simulink model "simulation"  (R2021b)
settings: Solver=VariableStepAuto  StartTime=0.0  StopTime=50  RelTol=1e-3
values from neighbouring files (symbols this model uses):
  g = 9.8    [script.m]
  l = 1    [script.m]
  m = 1    [script.m]
libraries: spsRMSLib x1
settings Model: Creator=mehdi  LastModifiedBy=mehdi

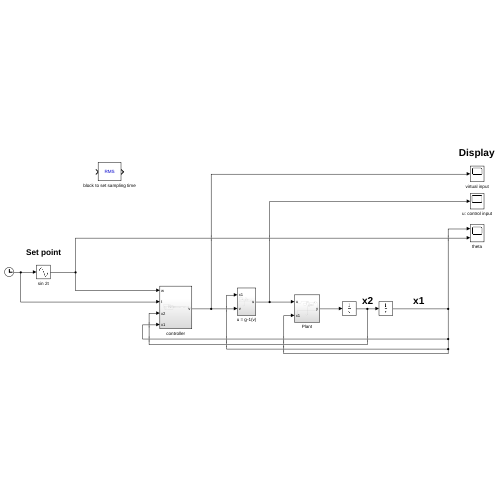
[thumbnail: Simulink's stored preview of the top-level diagram]
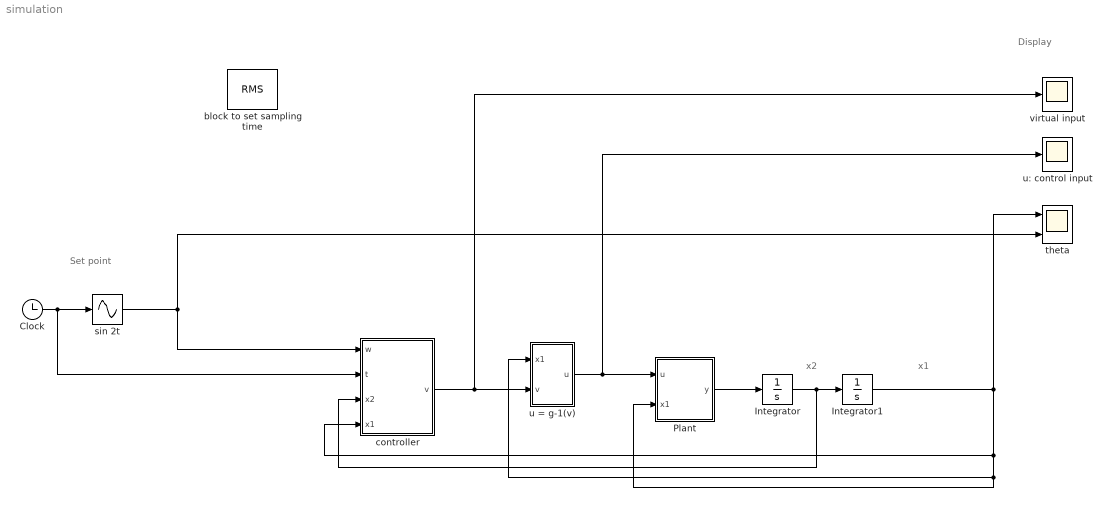
== system simulation ==
  note: Display
  note: x2
  note: Set point
  note: x1
  Clock : Clock
  Integrator : Integrator  ContinuousStateAttributes='omega'
  Integrator1 : Integrator  ContinuousStateAttributes='theta'
  Plant : Subsystem
  block to set sampling time : spsRMSLib/RMS  TrueRMS=on  Freq=60  RMSInit=120  Ts=0.001
  controller : Subsystem
  sin 2t : Sin  TimeSource=Use external signal  Frequency=2  SampleTime=0
  theta : Scope  NumInputPorts=2
  u = g-1(v) : Subsystem
  u: control input : Scope
  virtual input : Scope
  wires:
  Integrator/1 -> Integrator1/1, controller/3(x2)
  Integrator1/1 -> theta/1, Plant/2(x1), u = g-1(v)/1(x1), controller/4(x1)
  Clock/1 -> sin 2t/1, controller/2(t)
  sin 2t/1 -> theta/2, controller/1(w)
  controller/1(v) -> virtual input/1, u = g-1(v)/2(v)
  u = g-1(v)/1(u) -> u: control input/1, Plant/1(u)
  Plant/1(y) -> Integrator/1

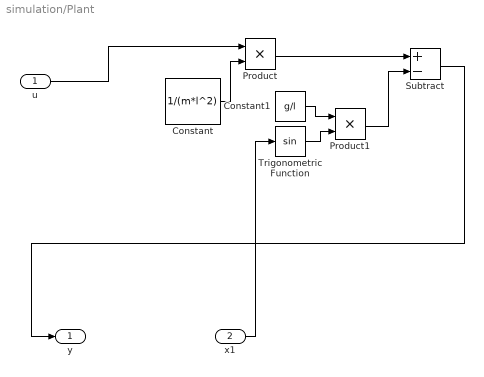
== system simulation/Plant ==
  u : Inport
  x1 : Inport  Port=2
  Constant : Constant  Value=1/(m*l^2)
  Constant1 : Constant  Value=g/l
  Product : Product
  Product1 : Product
  Subtract : Sum  Inputs=+-
  Trigonometric Function : Trigonometry
  y : Outport
  wires:
  u/1 -> Product/1
  Subtract/1 -> y/1
  Product/1 -> Subtract/1
  Constant1/1 -> Product1/1
  Constant/1 -> Product/2
  Product1/1 -> Subtract/2
  x1/1 -> Trigonometric Function/1
  Trigonometric Function/1 -> Product1/2

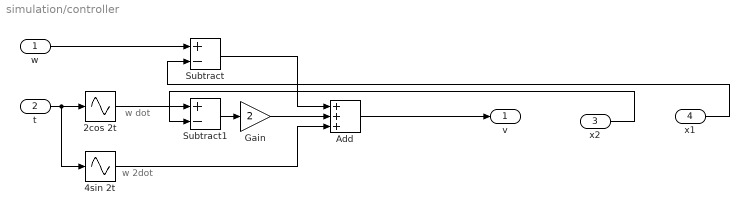
== system simulation/controller ==
  note: w 2dot
  note: w dot
  w : Inport
  t : Inport  Port=2
  x2 : Inport  Port=3
  x1 : Inport  Port=4
  2cos 2t : Sin  TimeSource=Use external signal  Amplitude=2  Frequency=2  Phase=90  SampleTime=0
  4sin 2t : Sin  TimeSource=Use external signal  Amplitude=-4  Frequency=2  SampleTime=0
  Add : Sum  Inputs=+++
  Gain : Gain  Gain=2
  Subtract : Sum  Inputs=+-
  Subtract1 : Sum  Inputs=+-
  v : Outport
  wires:
  4sin 2t/1 -> Add/3
  w/1 -> Subtract/1
  Subtract1/1 -> Gain/1
  t/1 -> 4sin 2t/1, 2cos 2t/1
  Gain/1 -> Add/2
  x1/1 -> Subtract/2
  Subtract/1 -> Add/1
  x2/1 -> Subtract1/2
  2cos 2t/1 -> Subtract1/1
  Add/1 -> v/1

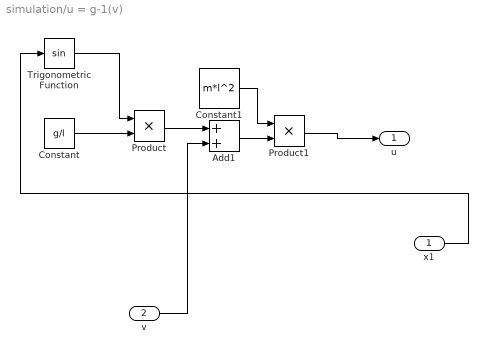
== system simulation/u = g-1(v) ==
  x1 : Inport
  v : Inport  Port=2
  Add1 : Sum
  Constant : Constant  Value=g/l
  Constant1 : Constant  Value=m*l^2
  Product : Product
  Product1 : Product
  Trigonometric Function : Trigonometry
  u : Outport
  wires:
  Product/1 -> Add1/1
  Add1/1 -> Product1/2
  v/1 -> Add1/2
  Product1/1 -> u/1
  Trigonometric Function/1 -> Product/1
  x1/1 -> Trigonometric Function/1
  Constant1/1 -> Product1/1
  Constant/1 -> Product/2
